simulink model "mySimScheme"  (R2021a)
settings: Solver=VariableStepAuto  StartTime=0.0  StopTime=10  RelTol=1e-3
model workspace (MAT data in the model file):
  firstWarning = 1
  originalScenarioChecksum = 'B59AFD355ACEE9D8A191C5001066B863'
values from neighbouring files (symbols this model uses):
  C = [ 1   0   0   0; 0   0   1   0]    [lpvGainScheduled.m]    (also in main.m = [1 0 0 0;0 1 0 0;0 0 1 0;0 0 0 1])
  Car = 80000    [main.m]
  K = W / X    [controlloreDstabilita.m]    (also in controlloreH2.m; controlloreHinfinito.m; controlloreL1.m; controlloreRobustoH2.m)
  Kv = ((lr*m)/(2*Caf*L))-((lf*m)/(2*Car*L))    (= 0.00176082089552)    [main.m]
  L = lf+lr    (= 2.68)    [main.m]
  lf = 1.1    [main.m]
  lr = 1.58    [main.m]
  m = 10.8    [lpvGainScheduled.m]    (also in main.m = 1573)
  Vx = 30    [main.m]
undefined symbols (not defined in the file or in its folder): driving
libraries: drivingscenarioandsensors x2, autolibshared x1
settings Model: EnablePacing=on  PacingRate=0.710000  Creator=nicol  LastModifiedBy=nicol

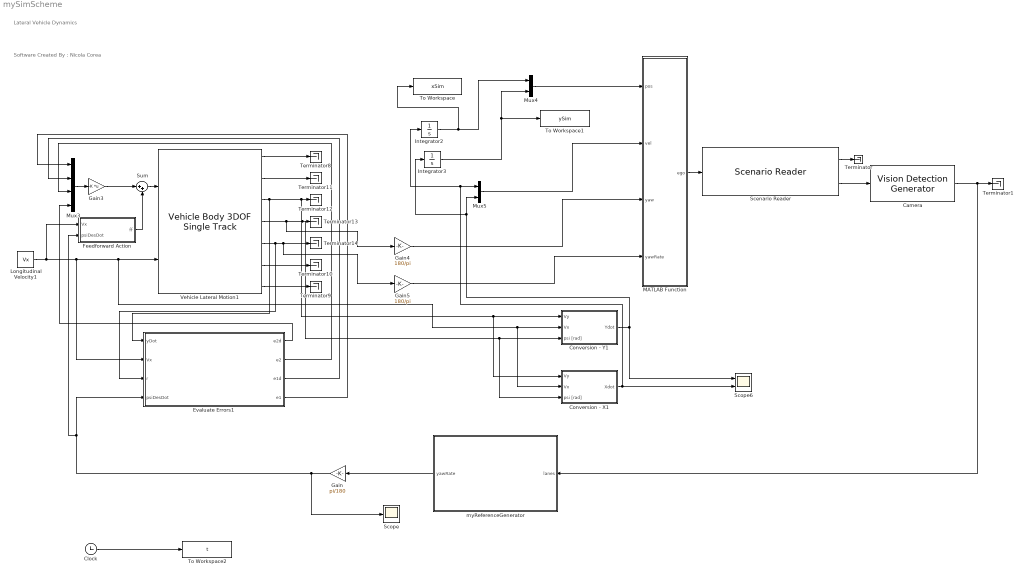
== system mySimScheme ==
  note: Software Created By : Nicola Corea
  note: Lateral Vehicle Dynamics
  Camera : drivingscenarioandsensors/Vision Detection Generator  SensorIndex=1  DetectorOutput=Lanes only  UpdateInterval=0.1  LaneUpdateInterval=0.1  SensorLocation=[3.7 0]  Height=1.1  Yaw=0  Pitch=1  Roll=0  BusNameSource=Auto  BusName=BusObjectDetections  BusName2Source=Auto  BusName2=BusLaneDetections  MaxNumDetectionsSource=Property  MaxNumDetections=50  MaxNumLanesSource=Property  MaxNumLanes=2  DetectionCoordinates=Ego Cartesian  SimulateUsing=Interpreted execution  MaxRange=15  BoundingBoxAccuracy=5  ProcessNoiseIntensity=5  MaxSpeed=100  MaxAllowedOcclusion=0.5  MinObjectImageSize=[15 15]  DetectionProbability=0.99  FalsePositivesPerImage=0  MinLaneImageSize=[20 3]  LaneBoundaryAccuracy=5  HasNoise=on  InitialSeedSource=Repeatable  InitialSeed=0  UsedSeed=0  ActorProfilesSource=From Scenario Reader block  ActorProfilesParameters=driving.internal.ActorProfilesParameters  ActorProfilesExpression=[struct('ActorID',1,'ClassID',1,'Length',4.7,'Width',1.8,'Height',1.4,'OriginOffset',[-1.35 0 0],'MeshVertices',[3.7 0.9 0.857439446366782;3.7 -0.9 0.857439446366782;3.7 -0.9 0.314878892733564;3.7 0.9 0.314878892733564;3.7 0.9 0.857439446366782;2.525 0.9 0.993079584775086;2.525 -0.9 0.993079584775086;3.7 -0.9 0.857439446366782;1.82 0.72 1.4;0.41 0.72 1.4;0.41 -0.72 1.4;1.82 -0.72 1.4;-0.295 0.9 0.993079584775086;-1 0.9 0.857439446366782;-1 -0.9 0.857439446366782;-0.295 -0.9 0.993079584775086;3.7 0.9 0.857439446366782;3.7 0.9 0.314878892733564;2.525 0.9 0.314878892733564;2.525 0.9 0.993079584775086;2.525 0.9 0.993079584775086;2.525 0.9 0.314878892733564;-0.295 0.9 0.314878892733564;-0.295 0.9 0.993079584775086;-0.295 0.9 0.993079584775086;-0.295 0.9 0.314878892733564;-1 0.9 0.355570934256055;-1 0.9 0.857439446366782;2.525 0.9 0.993079584775086;-0.295 0.9 0.993079584775086;0.41 0.72 1.4;1.82 0.72 1.4;3.7 -0.9 0.857439446366782;3.7 -0.9 0.314878892733564;2.525 -0.9 0.314878892733564;2.525 -0.9 0.993079584775086;2.525 -0.9 0.993079584775086;2.525 -0.9 0.314878892733564;-0.295 -0.9 0.314878892733564;-0.295 -0.9 0.993079584775086;-0.295 -0.9 0.993079584775086;-0.295 -0.9 0.314878892733564;-1 -0.9 0.355570934256055;-1 -0.9 0.857439446366782;2.525 -0.9 0.993079584775086;-0.295 -0.9 0.993079584775086;0.41 -0.72 1.4;1.82 -0.72 1.4;-0.295 0.9 0.993079584775086;-0.295 -0.9 0.993079584775086;0.41 -0.72 1.4;0.41 0.72 1.4;2.525 -0.9 0.993079584775086;1.82 -0.72 1.4;1.82 0.72 1.4;2.525 0.9 0.993079584775086;-1 0.9 0.857439446366782;-1 0.9 0.355570934256055;-1 -0.9 0.355570934256055;-1 -0.9 0.857439446366782;3.7 0.9 0.314878892733564;3.7 -0.9 0.314878892733564;-0.295 -0.9 0.314878892733564;-0.295 0.9 0.314878892733564;-0.295 0.9 0.314878892733564;-1 0.9 0.355570934256055;-1 -0.9 0.355570934256055;-0.295 -0.9 0.314878892733564;0 -0.63 0;0 -0.87 0;0.191030206995054 -0.63 0.0601365173421445;0.191030206995054 -0.87 0.0601365173421445;0.309093367795925 -0.63 0.217575963708927;0.309093367795925 -0.87 0.217575963708927;0.309093367795925 -0.63 0.412181821758201;0.309093367795925 -0.87 0.412181821758201;0.191030206995054 -0.63 0.569621268124983;0.191030206995054 -0.87 0.569621268124983;0 -0.63 0.629757785467128;0 -0.87 0.629757785467128;-0.191030206995054 -0.63 0.569621268124983;-0.191030206995054 -0.87 0.569621268124983;-0.309093367795925 -0.63 0.412181821758201;-0.309093367795925 -0.87 0.412181821758201;-0.309093367795925 -0.63 0.217575963708927;-0.309093367795925 -0.87 0.217575963708927;-0.191030206995054 -0.63 0.0601365173421445;-0.191030206995054 -0.87 0.0601365173421445;0 -0.63 0;0 -0.87 0;0 -0.63 0;0.191030206995054 -0.63 0.0601365173421445;0.309093367795925 -0.63 0.217575963708927;0.309093367795925 -0.63 0.412181821758201;0.191030206995054 -0.63 0.569621268124983;0 -0.63 0.629757785467128;-0.191030206995054 -0.63 0.569621268124983;-0.309093367795925 -0.63 0.412181821758201;-0.309093367795925 -0.63 0.217575963708927;-0.191030206995054 -0.63 0.0601365173421445;0 -0.87 0;0.191030206995054 -0.87 0.0601365173421445;0.309093367795925 -0.87 0.217575963708927;0.309093367795925 -0.87 0.412181821758201;0.191030206995054 -0.87 0.569621268124983;0 -0.87 0.629757785467128;-0.191030206995054 -0.87 0.569621268124983;-0.309093367795925 -0.87 0.412181821758201;-0.309093367795925 -0.87 0.217575963708927;-0.191030206995054 -0.87 0.0601365173421445;0 0.87 0;0 0.63 0;0.191030206995054 0.87 0.0601365173421445;0.191030206995054 0.63 0.0601365173421445;0.309093367795925 0.87 0.217575963708927;0.309093367795925 0.63 0.217575963708927;0.309093367795925 0.87 0.412181821758201;0.309093367795925 0.63 0.412181821758201;0.191030206995054 0.87 0.569621268124983;0.191030206995054 0.63 0.569621268124983;0 0.87 0.629757785467128;0 0.63 0.629757785467128;-0.191030206995054 0.87 0.569621268124983;-0.191030206995054 0.63 0.569621268124983;-0.309093367795925 0.87 0.412181821758201;-0.309093367795925 0.63 0.412181821758201;-0.309093367795925 0.87 0.217575963708927;-0.309093367795925 0.63 0.217575963708927;-0.191030206995054 0.87 0.0601365173421445;-0.191030206995054 0.63 0.0601365173421445;0 ...(+3718 chars)],'MeshFaces',[1 2 3;3 4 1;5 6 7;7 8 5;9 10 11;11 12 9;13 14 15;15 16 13;17 18 19;19 20 17;21 22 23;23 24 21;25 26 27;27 28 25;29 30 31;31 32 29;33 34 35;35 36 33;37 38 39;39 40 37;41 42 43;43 44 41;45 46 47;47 48 45;49 50 51;51 52 49;53 54 55;55 56 53;57 58 59;59 60 57;61 62 63;63 64 61;65 66 67;67 68 65;69 71 72;72 70 69;71 73 74;74 72 71;73 75 76;76 74 73;75 77 78;78 76 75;77 79 80;80 78 77;79 81 82;82 80 79;81 83 84;84 82 81;83 85 86;86 84 83;85 87 88;88 86 85;87 89 90;90 88 87;91 92 93;91 93 94;91 94 95;91 95 96;91 96 97;91 97 98;91 98 99;91 99 100;101 102 103;101 103 104;101 104 105;101 105 106;101 106 107;101 107 108;101 108 109;101 109 110;111 113 114;114 112 111;113 115 116;116 114 113;115 117 118;118 116 115;117 119 120;120 118 117;119 121 122;122 120 119;121 123 124;124 122 121;123 125 126;126 124 123;125 127 128;128 126 125;127 129 130;130 128 127;129 131 132;132 130 129;133 134 135;133 135 136;133 136 137;133 137 138;133 138 139;133 139 140;133 140 141;133 141 142;143 144 145;143 145 146;143 146 147;143 147 148;143 148 149;143 149 150;143 150 151;143 151 152;153 155 156;156 154 153;155 157 158;158 156 155;157 159 160;160 158 157;159 161 162;162 160 159;161 163 164;164 162 161;163 165 166;166 164 163;165 167 168;168 166 165;167 169 170;170 168 167;169 171 172;172 170 169;171 173 174;174 172 171;175 176 177;175 177 178;175 178 179;175 179 180;175 180 181;175 181 182;175 182 183;175 183 184;185 186 187;185 187 188;185 188 189;185 189 190;185 190 191;185 191 192;185 192 193;185 193 194;195 197 198;198 196 195;197 199 200;200 198 197;199 201 202;202 200 199;201 203 204;204 202 201;203 205 206;206 204 203;205 207 208;208 206 205;207 209 210;210 208 207;209 211 212;212 210 209;211 213 214;214 212 211;213 215 216;216 214 213;217 218 219;217 219 220;217 220 221;217 221 222;217 222 223;217 223 224;217 224 225;217 225 226;227 228 229;227 229 230;227 230 231;227 231 232;227 232 233;227 233 234;227 234 235;227 235 236],'RCSPattern',[10 10;10 10],'RCSAzimuthAngles',[-180 180],'RCSElevationAngles',[-90 90])]  Intrinsics=driving.internal.cameraIntrinsics('FocalLength',[1814.81018227767 1814.81018227767],'PrincipalPoint',[320 240],'ImageSize',[480 640],'RadialDistortion',[0 0],'TangentialDistortion',[0 0],'Skew',0)
  Clock : Clock
  Conversion - X1 : Subsystem
  Conversion - Y1 : Subsystem
  Evaluate Errors1 : Subsystem
  Feedforward Action : Subsystem
  Gain : Gain  Gain=pi/180
  Gain3 : Gain  Gain=-K  Multiplication=Matrix(K*u) (u vector)
  Gain4 : Gain  Gain=180/pi
  Gain5 : Gain  Gain=180/pi
  Integrator2 : Integrator  InitialCondition=-51.6000
  Integrator3 : Integrator  InitialCondition=-45.3000
  Longitudinal Velocity1 : Constant  Value=Vx
  MATLAB Function : MATLAB Function  TreatAsAtomicUnit=on
  Mux3 : Mux
  Mux4 : Mux  Inputs=2
  Mux5 : Mux  Inputs=2
  Scenario Reader : drivingscenarioandsensors/Scenario Reader  ScenarioSource=From file  ScenarioFileName=C:\Users\nicol\Desktop\ProgettoFinale-NicolaCorea\Modulo2\DrivingScenarioLateral\simulationScenario.mat  ScenarioVariableName=scenario  OutputCoordinateSystem=Vehicle coordinates  EgoVehicleSource=Input port  EgoVehicleActorID=1  OrientVehiclesOnRoad=off  OutputEgoVehiclePose=off  SampleTime=0.1  LaneBoundaryOutput=Ego vehicle lane boundaries  LaneBoundaryDistance=linspace(-20, 20, 101)  LaneBoundaryLocation=Center of lane markings  BusNameSource=Auto  BusName=BusActors  BusNumActorsSource=Scenario  BusNumActors=100  BusName2Source=Auto  BusName2=BusLaneBoundaries  BusNumLaneBoundariesSource=Scenario  BusNumLaneBoundaries=10  BusName3Source=Auto  BusName3=BusEgoActor  ShowCoordinateLabels=on  SimulateUsing=Interpreted execution
  Scope : Scope
  Scope6 : Scope  NumInputPorts=2
  Sum : Sum  Inputs=|++
  Terminator{,1,8..14} (9 alike) : Terminator
  To Workspace : ToWorkspace  VariableName=xSim  SampleTime=0.1
      settings: Save2DSignal=2-D array (concatenate along first dimension)
  To Workspace1 : ToWorkspace  VariableName=ySim  SampleTime=0.1
      settings: Save2DSignal=2-D array (concatenate along first dimension)
  To Workspace2 : ToWorkspace  VariableName=t  SampleTime=0.1
      settings: Save2DSignal=2-D array (concatenate along first dimension)
  Vehicle Lateral Motion1 : autolibshared/Vehicle Body 3DOF Single Track  trackMode=Single (bicycle)  inputMode=External longitudinal velocity  frontSteerMode=on  rearSteerMode=off  windMode=off  muMode=off  extFMode=off  extMMode=off  htchFMode=off  htchMMode=off  extXo=off  extpsio=off  extxdoto=off  extro=off  extYo=off  extTamb=off  extydoto=off  aMode=2  NF=2  NR=2  m=m  a=lf  b=lr  h=0.35  dh=1  hh=0.2  X_o=0  xdot_o=0  CalphaMode=off  sigmaMode=on  d=0  hl=0  w=[1.4,1.4]  Cy_f=Caf  Cy_r=Car  sigma_f=.1  sigma_r=.1  alpha_f_brk=[-.1 .1]  Cy_f_data=[-9e3 9e3]  alpha_r_brk=[-.1 .1]  Cy_r_data=[-9e3 9e3]  Y_o=0  ydot_o=0  Izz=Iz  psi_o=0  r_o=0  Af=2  Cd=.3  Cl=.1  Cpm=.1  beta_w=[0:0.01:0.3]  Cs=[0:0.03:0.9]  Cym=[0:0.01:0.3]  Pabs=101325  Tair=273  g=9.81  mu=1  xdot_tol=.01  Fznom=5000  Fxtire_sat=7e4  Fytire_sat=7e4  longOff=0  latOff=0  vertOff=0  wrapAng=off
      settings: SourceProductBaseCode=PW,DR,MT,UV,VE
  myReferenceGenerator : MATLAB Function  TreatAsAtomicUnit=on
  wires:
  Scenario Reader/2 -> Camera/1
  Scenario Reader/1 -> Terminator/1
  Camera/1 -> myReferenceGenerator/1(lanes), Terminator1/1
  Vehicle Lateral Motion1/4 -> Gain4/1, Conversion - X1/3(psi [rad]), Conversion - Y1/3(psi [rad]), Terminator13/1
  Vehicle Lateral Motion1/5 -> Evaluate Errors1/3(r), Gain5/1, Terminator14/1
  Mux4/1 -> MATLAB Function/1(pos)
  Vehicle Lateral Motion1/1 -> Terminator8/1
  Vehicle Lateral Motion1/3 -> Evaluate Errors1/1(yDot), Conversion - X1/1(Vy), Conversion - Y1/1(Vy), Terminator12/1
  Vehicle Lateral Motion1/2 -> Terminator11/1
  Evaluate Errors1/4(e1) -> Mux3/1
  Mux3/1 -> Gain3/1
  Vehicle Lateral Motion1/6 -> Terminator10/1
  Mux5/1 -> MATLAB Function/2(vel)
  Vehicle Lateral Motion1/7 -> Terminator9/1
  Evaluate Errors1/3(e1d) -> Mux3/2
  Evaluate Errors1/1(e2d) -> Mux3/4
  Gain4/1 -> MATLAB Function/3(yaw)
  Evaluate Errors1/2(e2) -> Mux3/3
  Integrator3/1 -> To Workspace1/1, Mux4/2
  Integrator2/1 -> To Workspace/1, Mux4/1
  Gain5/1 -> MATLAB Function/4(yawRate)
  Longitudinal Velocity1/1 -> Feedforward Action/1(Vx), Evaluate Errors1/2(Vx), Conversion - X1/2(Vx), Conversion - Y1/2(Vx), Vehicle Lateral Motion1/2
  MATLAB Function/1(ego) -> Scenario Reader/1
  Conversion - Y1/1(Ydot) -> Integrator3/1, Mux5/2, Scope6/1
  Conversion - X1/1(Xdot) -> Mux5/1, Integrator2/1, Scope6/2
  myReferenceGenerator/1(yawRate) -> Gain/1
  Gain/1 -> Scope/1, Feedforward Action/2(psiDesDot), Evaluate Errors1/4(psiDesDot)
  Clock/1 -> To Workspace2/1
  Gain3/1 -> Sum/1
  Sum/1 -> Vehicle Lateral Motion1/1
  Feedforward Action/1(ff) -> Sum/2

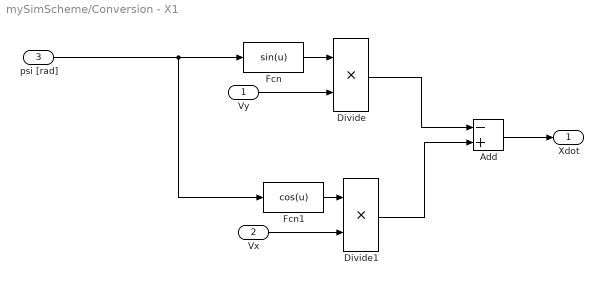
== system mySimScheme/Conversion - X1 ==
  Vy : Inport
  Vx : Inport  Port=2
  psi [rad] : Inport  Port=3
  Add : Sum  Inputs=-+
  Divide : Product  Inputs=**
  Divide1 : Product  Inputs=**
  Fcn : Fcn  Expr=sin(u)
  Fcn1 : Fcn  Expr=cos(u)
  Xdot : Outport
  wires:
  psi [rad]/1 -> Fcn/1, Fcn1/1
  Add/1 -> Xdot/1
  Divide1/1 -> Add/2
  Vx/1 -> Divide1/2
  Fcn1/1 -> Divide1/1
  Divide/1 -> Add/1
  Vy/1 -> Divide/2
  Fcn/1 -> Divide/1

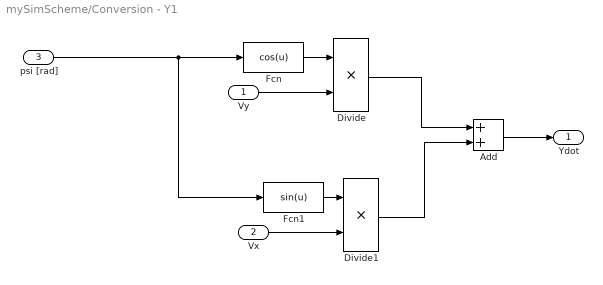
== system mySimScheme/Conversion - Y1 ==
  Vy : Inport
  Vx : Inport  Port=2
  psi [rad] : Inport  Port=3
  Add : Sum
  Divide : Product  Inputs=**
  Divide1 : Product  Inputs=**
  Fcn : Fcn  Expr=cos(u)
  Fcn1 : Fcn  Expr=sin(u)
  Ydot : Outport
  wires:
  Fcn/1 -> Divide/1
  Vy/1 -> Divide/2
  Divide/1 -> Add/1
  Fcn1/1 -> Divide1/1
  Vx/1 -> Divide1/2
  Divide1/1 -> Add/2
  Add/1 -> Ydot/1
  psi [rad]/1 -> Fcn1/1, Fcn/1

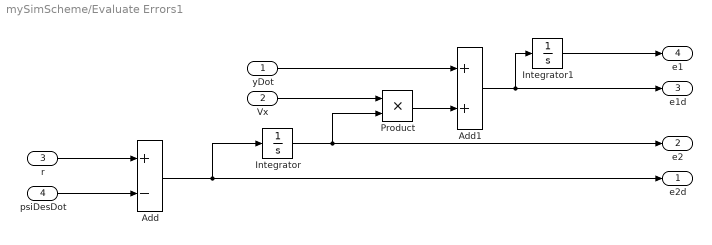
== system mySimScheme/Evaluate Errors1 ==
  yDot : Inport
  Vx : Inport  Port=2
  r : Inport  Port=3
  psiDesDot : Inport  Port=4
  Add : Sum  Inputs=+-
  Add1 : Sum
  Integrator : Integrator
  Integrator1 : Integrator
  Product : Product
  e2d : Outport
  e2 : Outport  Port=2
  e1d : Outport  Port=3
  e1 : Outport  Port=4
  wires:
  Product/1 -> Add1/2
  Integrator/1 -> e2/1, Product/2
  Add1/1 -> e1d/1, Integrator1/1
  Vx/1 -> Product/1
  Add/1 -> e2d/1, Integrator/1
  Integrator1/1 -> e1/1
  r/1 -> Add/1
  yDot/1 -> Add1/1
  psiDesDot/1 -> Add/2

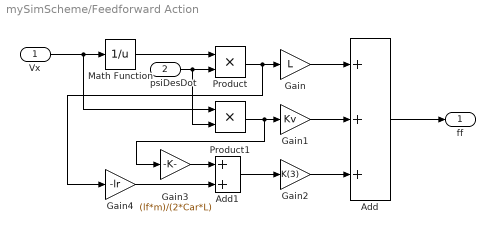
== system mySimScheme/Feedforward Action ==
  Vx : Inport
  psiDesDot : Inport  Port=2
  Add : Sum  Inputs=+++
  Add1 : Sum
  Gain : Gain  Gain=L
  Gain1 : Gain  Gain=Kv
  Gain2 : Gain  Gain=K(3)
  Gain3 : Gain  Gain=(lf*m)/(2*Car*L)
  Gain4 : Gain  Gain=-lr
  Math Function : Math  Operator=reciprocal  SaturateOnIntegerOverflow=on
  Product : Product
  Product1 : Product
  ff : Outport
  wires:
  Add/1 -> ff/1
  Gain/1 -> Add/1
  Product/1 -> Gain4/1, Gain/1
  Math Function/1 -> Product/1
  Vx/1 -> Product1/1, Math Function/1
  psiDesDot/1 -> Product1/2, Product/2
  Gain1/1 -> Add/2
  Product1/1 -> Gain3/1, Gain1/1
  Gain2/1 -> Add/3
  Add1/1 -> Gain2/1
  Gain3/1 -> Add1/1
  Gain4/1 -> Add1/2

== matlab function mySimScheme/myReferenceGenerator ==
  data: lanes input; yawRate output
function yawRate  = getReference(lanes)
% This Function Generates yawRate reference From Lanes Detections
yawRate = 0;
% Get Lanes Detected
left              = lanes.LaneBoundaries(1);
right             = lanes.LaneBoundaries(2);
% Controlling Which Lanes are Detected
vLeft             = left.Strength;
vRight            = right.Strength;
% Control Visibility of Lanes
if (vLeft > 0 && vRight > 0)
    % Both Lanes Are Detected
    laneDepartureFromLeft = abs(left.LateralOffset);
    laneDepartureFromRight= abs(right.LateralOffset);
    % Evaluta Distance Ego Vehicle
    if(laneDepartureFromLeft > laneDepartureFromRight)
        % Much closed to Right Lane
        curvature  = right.Curvature * right.CurveLength;
        % Control The Orientation
        if(curvature >= 0)
                yawRate    = 0.15*(curvature/0.1);
        else
                yawRate    = -0.15*(curvature/0.1);
        end
    elseif(laneDepartureFromLeft < laneDepartureFromRight)
        % Much closed to Left Lane
        curvature  = left.Curvature * left.CurveLength;
        % Control The Orientation
        if(curvature >= 0)
                yawRate    = -0.15*(curvature/0.1);
        else
                yawRate    =  0.15*(curvature/0.1);
        end
    else
        % Go forward -> same distance from both
        yawRate    = 0;
    end
elseif (vLeft > 0)
    % Only Left Lane
    leftCurvature = left.Curvature * left.CurveLength;     % meter
    % Evaluate An Approximation to yaw Angle
    curvature     = (-1)*leftCurvature;
    % Control Of Curvature
    if(curvature >= 0)
          yawRate = (curvature / 0.1)*-0.15;
    else
          yawRate = (curvature / 0.1)*0.15;
    end
elseif (vRight > 0)
    % Only Right Lane
    rightCurvature= right.Curvature * right.CurveLength;   % meter
    % Evaluate An Approximation to yaw Angle
    curvature     = rightCurvature;
    % Control Of Curvature
    if(curvature >= 0)
          yawRate = (curvature / 0.1)*0.15;
    else
          yawRate = (curvature / 0.1)*-0.15;
    end
end
end

== matlab function mySimScheme/MATLAB Function ==
  data: pos input; ego output Bus: BusActors1Actors; vel input; yaw input; yawRate input
function ego = packEgo(pos,vel,yaw,yawRate)
ego          = struct('ActorID',1,...
                      'Position',[pos(1) pos(2) 0],...
                      'Velocity',[vel(1) vel(2) 0],...
                      'Roll',0,...
                      'Pitch',0,...
                      'Yaw',yaw,...
                      'AngularVelocity',[0 0 yawRate]);
end
